simulink model "ofdmexample1"  (R2017a)
settings: Solver=FixedStepDiscrete  StartTime=0.0  StopTime=0.1  RelTol=1e-3
PostLoadFcn:
  | prm80216d.blkh = []; prm80216d.action = 'init';
  | commwman80216d_init(prm80216d.blkh, prm80216d.action);
  | if isempty(ans), clear ans; end
StartFcn:
  | if isempty(ans), clear ans; end
undefined symbols (not defined in the file): magnitude
libraries: commwman80216d_lib x25, dspsigops x8, commcnvcod2 x7, dspindex x4, commdigbbndpm3 x2, commblksprivate x1, commofdm x1, commsdrhw_v2 x1
Description:
  | IEEE 802.16-2004 WirelessMAN-OFDM PHY Downlink model
settings Model: FPTRunName=Active  ExtModeAutoUpdateStatusClock=off  Creator=The MathWorks, Inc.  LastModifiedBy=max
settings DataIOCC: LimitDataPoints=on  SaveFormat=Array
settings OptimizationCC: ExpressionDepthLimit=2147483647  InitFltsAndDblsToZero=on  EfficientMapNaN2IntZero=off  LifeSpan=inf
settings DebuggingCC: UnderspecifiedInitializationDetection=Classic  MergeDetectMultiDrivingBlocksExec=none  FcnCallInpInsideContextMsg=warning  AllowSymbolicDim=off  StateNameClashWarn=warning  SFUnexpectedBacktrackingDiag=warning  SFNoUnconditionalDefaultTransitionDiag=warning  SFExecutionAtInitializationDiag=none
settings HardwareCC: ProdBitPerPointer=32  ProdBitPerSizeT=32  ProdBitPerPtrDiffT=32  ProdLargestAtomicFloat=None  ProdIntDivRoundTo=Undefined  ProdEndianess=Unspecified  ProdWordSize=32  ProdHWDeviceType=32-bit Generic
settings ModelReferenceCC: PropagateSignalLabelsOutOfModel=off
settings RTWCC: RetainRTWFile=on
settings GRTTargetCC: TargetFcnLib=ansi_tfl_tmw_new.mat  TargetLangStandard=C89/C90 (ANSI)  GeneratePreprocessorConditionals=Disable all  CombineOutputUpdateFcns=off  GRTInterface=on
settings ConfigComp: CovMetricSettings=dw  CovHtmlReporting=on  CovSaveCumulativeToWorkspaceVar=on  CovSaveSingleToWorkspaceVar=on  CovExternalEMLEnable=off  CovSFcnEnable=off

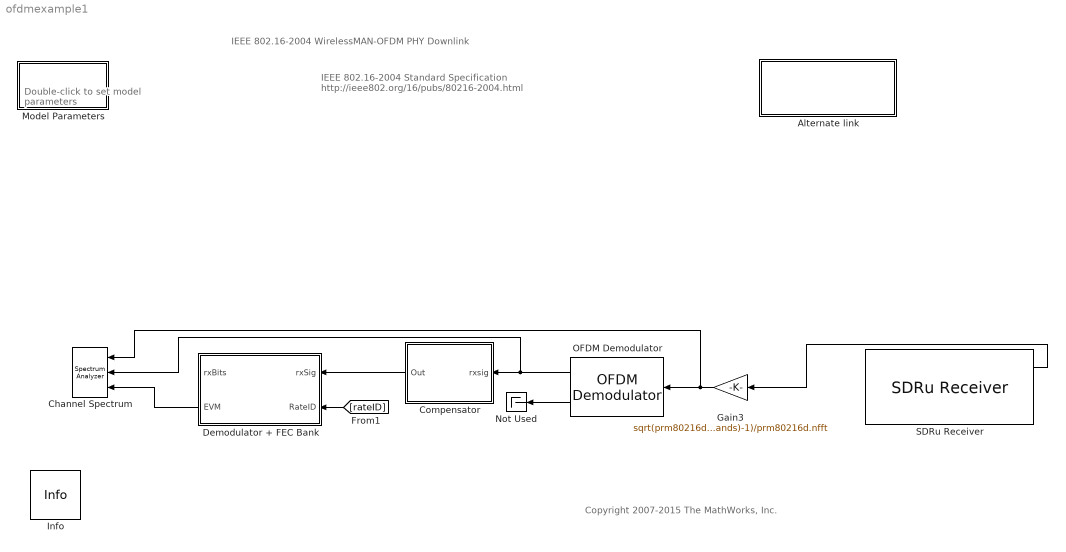
== system ofdmexample1 ==
  note: IEEE 802.16-2004 WirelessMAN-OFDM PHY Downlink
  note: Double-click to
      | set model parameters
  note: IEEE 802.16-2004 Standard Specification
      | http://ieee802.org/16/pubs/80216-2004.html
  note: Copyright 2007-2015 The MathWorks, Inc.
  Alternate link : Subsystem
      settings: OpenFcn=commwman80216dstbc;
      mask Display: disp('Double-click to open\n link model with\nSpace-Time Block Coding');
  Channel Spectrum : SpectrumAnalyzer  NumInputPorts=3
  Compensator : Subsystem
      mask Display: disp('Gain & Phase\nCompensator');
  Demodulator + FEC Bank : Subsystem
      mask Display: disp('Demodulator\n& FEC Bank');
  Gain3 : Gain  Gain=sqrt(prm80216d.nfft-sum(prm80216d.guardBands)-1)/prm80216d.nfft
  Info : commblksprivate/Info  SystemSampleTime=-1
      settings: SourceProductName=Communications System Toolbox  SourceProductBaseCode=CM
  Model Parameters : Subsystem  mask(Model Parameters){chanBW=3.5, numSym=1, g=1/8, nonlinCtrl=Disabled, dpdCtrl=Disabled, thresh=[4 10 12 19 22 28]}
      mask prompts: chanBW "Channel bandwidth (MHz):"; numSym "Number of OFDM symbols per burst:"; g "Cyclic prefix factor (G):"; nonlinCtrl "Amplifier nonlinearity:"; dpdCtrl "Digital pre-distortion:"; thresh "Low SNR thresholds for rate control (dB):"
      mask help: Specifies model parameters for a simulation run.
      mask init:
      | numPreSym = 1; % number of preamble OFDM symbols
      | 
      | % If the nonlinearity is turned off, then turn off the digital
      | % pre-distortion
      | if nonlinCtrl == 1  % disabled
      |     dpdCtrl = 1;
      | end
      | 
      | myException = commwman80216d_init(gcbh, 'init', chanBW, ...
      |     numSym, numPreSym, g, thresh);
      | 
      | if ~isempty(myException)
      |     errordlg(myException.msg);
      | end
      mask Help: helpview(commdhelp);
      mask TypeOptions g: 1/4 | 1/8 | 1/16 | 1/32
      mask TypeOptions nonlinCtrl: Disabled | Moderate (correctable by pre-distortion) | Severe (uncorrectable by pre-distortion)
      mask Callback nonlinCtrl: commwman80216d_init(gcbh, 'cbShowHidePreDistortion');
      mask TypeOptions dpdCtrl: Disabled | Enabled
      mask Display: disp('Model\nParameters');
  Not Used : Terminator
  OFDM Demodulator : commofdm/OFDM Demodulator  FFTLength=prm80216d.nfft  NumGuardBandCarriers=prm80216d.guardBands  RemoveDCCarrier=on  PilotOutputPort=on  PilotCarrierIndices=prm80216d.pilotIndices + prm80216d.nfft/2 + 1  CyclicPrefixLength=prm80216d.CPLen  NumSymbols=prm80216d.totOFDMSym  NumReceiveAntennas=1  SimulateUsing=Interpreted execution
      settings: SourceProductName=Communications System Toolbox  SourceProductBaseCode=CM
  SDRu Receiver : commsdrhw_v2/SDRu Receiver  SourceLibraryInfo="This block requires <a href=\"http://www.mathworks.com/hardware-support/usrp.html\">Communications System Toolbox Support Package for USRP Radio</a>"  rxtx=rx  platform=B210  USRP2_IP='192.168.10.2'  USRP_IP_X300='192.168.10.2'  USRP_IP_X310='192.168.10.2'  USRP_serialNumB200=''  USRP_serialNumB210='30D0D1D'  ChannelMapping=1  centerFrequency=2.484e9  centerFrequencySrc=Dialog  loOffset=0  loOffsetSrc=Dialog  PPSSource=Internal  clockSource=Internal  masterClkRateB200=32e6  masterClkRateB210=8e6  masterClkRateX300=200e6  masterClkRateX310=200e6  masterClkRateParam=8000000  gain=40  gainSrc=Dialog  decimInterpSrc=Dialog  decimInterp=512  TransportDataType=int16  USRP2_IP_NUM=[51 48 68 48 68 49 68]  frameLength=362  outputDatatype=Same as transport data type  overrunUnderrunPort=off  sampleTime=1/15625  HOST_DATA_PORT=0  HOST_CONTROL_PORT=0  USRP2_DATA_PORT=0  USRP2_CONTROL_PORT=0  bufferMode=Continuous streaming  EnableBurstMode=off  NumFramesInBurst=100  USRP_ID='30D0D1D'
      settings: SourceProductName=Communications System Toolbox Support Package for USRP(R) Radio  SourceProductBaseCode=USRP
  wires:
  [rateID] -> Demodulator + FEC Bank/2(RateID)
  Gain3/1 -> Channel Spectrum/1, OFDM Demodulator/1
  OFDM Demodulator/1 -> Channel Spectrum/2, Compensator/1(rxsig)
  OFDM Demodulator/2 -> Not Used/1
  Compensator/1(Out) -> Demodulator + FEC Bank/1(rxSig)
  Demodulator + FEC Bank/2(EVM) -> Channel Spectrum/3
  SDRu Receiver/1 -> Gain3/1

== system ofdmexample1/Alternate link ==

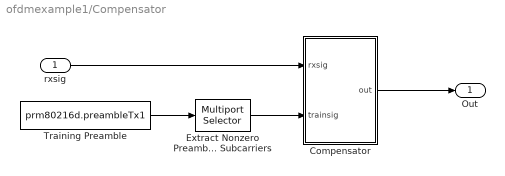
== system ofdmexample1/Compensator ==
  rxsig : Inport
  Compensator : Subsystem
      mask init:
      | a = [1:100; 1:100];
      mask Display: disp('Gain & Phase\nCompensator')
  Extract Nonzero Preamble Subcarriers : dspindex/Multiport Selector  rowsOrCols=Rows  idxCellArray=prm80216d.nonzeroPreambleIdxTx1  idxErrMode=Clip Index
  Training Preamble : Constant  Value=prm80216d.preambleTx1  VectorParams1D=off
  Out : Outport
  wires:
  Training Preamble/1 -> Extract Nonzero Preamble Subcarriers/1
  rxsig/1 -> Compensator/1(rxsig)
  Compensator/1(out) -> Out/1
  Extract Nonzero Preamble Subcarriers/1 -> Compensator/2(trainsig)

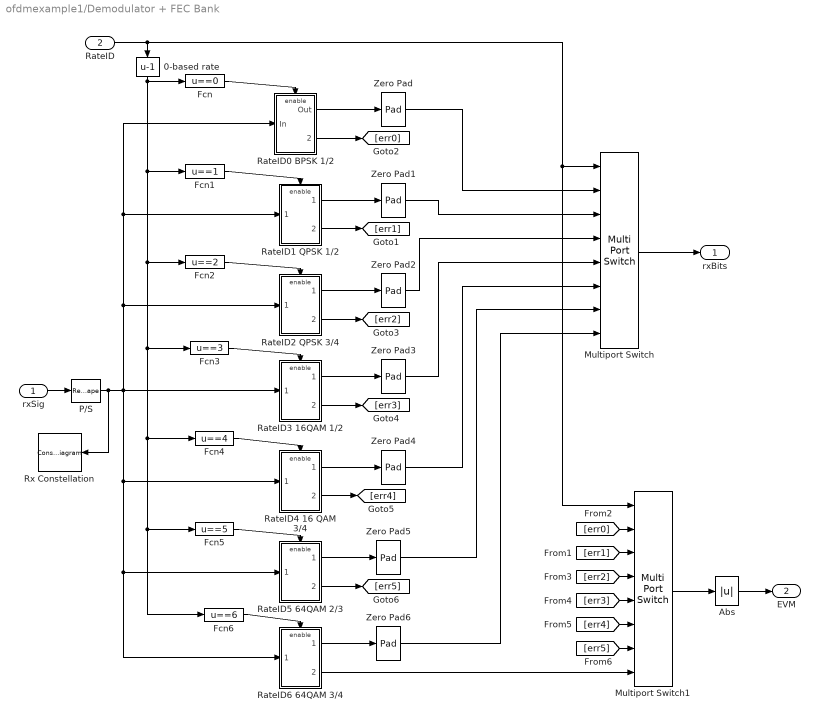
== system ofdmexample1/Demodulator + FEC Bank ==
  rxSig : Inport
  RateID : Inport  Port=2
  0-based rate : Bias  Bias=-1
  Abs : Abs  SaturateOnIntegerOverflow=on
  Fcn : Fcn  Expr=u==0
  Fcn1 : Fcn  Expr=u==1
  Fcn2 : Fcn  Expr=u==2
  Fcn3 : Fcn  Expr=u==3
  Fcn4 : Fcn  Expr=u==4
  Fcn5 : Fcn  Expr=u==5
  Fcn6 : Fcn  Expr=u==6
  Multiport Switch : MultiPortSwitch  Inputs=7  SaturateOnIntegerOverflow=on
  Multiport Switch1 : MultiPortSwitch  Inputs=7  SaturateOnIntegerOverflow=on
  P/S : Reshape  OutputDimensionality=Column vector (2-D)  OutputDimensions=[prm80216d.numDataSym, prm80216d.numOFDMSymbols]
  RateID0 BPSK 1/2 : Subsystem
  RateID1 QPSK 1/2 : Subsystem
  RateID2 QPSK 3/4 : Subsystem
  RateID3 16QAM 1/2 : Subsystem
  RateID4 16 QAM 3/4 : Subsystem
  RateID5 64QAM 2/3 : Subsystem
  RateID6 64QAM 3/4 : Subsystem
  Rx Constellation : ConstellationDiagram  Tag=ScatterPlot
  Zero Pad{,1..6} (7 alike) : dspsigops/Pad  padAlong=Columns  dimsToPad=1  valSrc=Specify via dialog  padVal=0  spec=Output size  padNumOutRowsSpecMethod=User-specified  numOutRows=prm80216d.maxUncBitsPerBlk*prm80216d.numOFDMSymbols  padNumOutColsSpecMethod=User-specified  numOutCols=1  isVarDimsMode=off  padBeginning=0  padEnd=0  outSizeMode=User-specified  outSize=1  padSigAt=End  trunc_flag=None  roundingMode=Floor  overflowMode=off  truncOrWrapMode=Truncate  wrap_flag=None
      settings: AttributesFormatString=\n  SourceProductName=DSP System Toolbox  SourceProductBaseCode=DS
  rxBits : Outport
  EVM : Outport  Port=2
  wires:
  RateID/1 -> Multiport Switch/1, Multiport Switch1/1, 0-based rate/1
  Multiport Switch/1 -> rxBits/1
  RateID0 BPSK 1/2/1(Out) -> Zero Pad/1
  RateID1 QPSK 1/2/1(Out1) -> Zero Pad1/1
  RateID2 QPSK 3/4/1(Out2) -> Zero Pad2/1
  RateID3 16QAM 1/2/1(Out3) -> Zero Pad3/1
  RateID4 16 QAM 3/4/1(Out4) -> Zero Pad4/1
  RateID5 64QAM 2/3/1(Out5) -> Zero Pad5/1
  RateID6 64QAM 3/4/1(Out6) -> Zero Pad6/1
  Fcn/1 -> RateID0 BPSK 1/2/Enable
  Fcn1/1 -> RateID1 QPSK 1/2/Enable
  Fcn2/1 -> RateID2 QPSK 3/4/Enable
  Fcn3/1 -> RateID3 16QAM 1/2/Enable
  Fcn4/1 -> RateID4 16 QAM 3/4/Enable
  Fcn5/1 -> RateID5 64QAM 2/3/Enable
  Fcn6/1 -> RateID6 64QAM 3/4/Enable
  Zero Pad/1 -> Multiport Switch/2
  Zero Pad2/1 -> Multiport Switch/4
  Zero Pad3/1 -> Multiport Switch/5
  Zero Pad4/1 -> Multiport Switch/6
  Zero Pad5/1 -> Multiport Switch/7
  Zero Pad6/1 -> Multiport Switch/8
  Multiport Switch1/1 -> Abs/1
  RateID6 64QAM 3/4/2(symerr) -> Multiport Switch1/8
  Abs/1 -> EVM/1
  0-based rate/1 -> Fcn/1, Fcn1/1, Fcn2/1, Fcn3/1, Fcn4/1, Fcn5/1, Fcn6/1
  RateID0 BPSK 1/2/2(symerr) -> [err0]
  RateID1 QPSK 1/2/2(symerr) -> [err1]
  RateID2 QPSK 3/4/2(symerr) -> [err2]
  RateID3 16QAM 1/2/2(symerr) -> [err3]
  RateID4 16 QAM 3/4/2(symerr) -> [err4]
  RateID5 64QAM 2/3/2(symerr) -> [err5]
  [err0] -> Multiport Switch1/2
  [err1] -> Multiport Switch1/3
  [err2] -> Multiport Switch1/4
  [err3] -> Multiport Switch1/5
  [err4] -> Multiport Switch1/6
  [err5] -> Multiport Switch1/7
  Zero Pad1/1 -> Multiport Switch/3
  rxSig/1 -> P/S/1
  P/S/1 -> Rx Constellation/1, RateID4 16 QAM 3/4/1(In4), RateID5 64QAM 2/3/1(In5), RateID6 64QAM 3/4/1(In6), RateID0 BPSK 1/2/1(In), RateID1 QPSK 1/2/1(In1), RateID2 QPSK 3/4/1(In2), RateID3 16QAM 1/2/1(In3)

== system ofdmexample1/Model Parameters ==
  note: This subsystem is empty.
      | It is used for setting parameter values (in the mask).

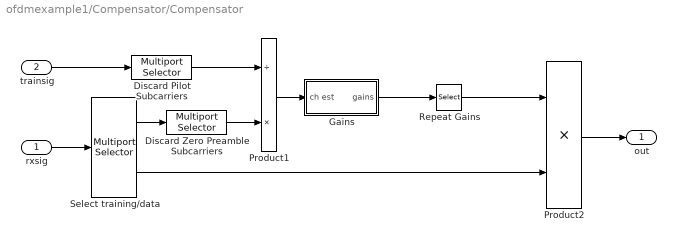
== system ofdmexample1/Compensator/Compensator ==
  rxsig : Inport
  trainsig : Inport  Port=2
  Discard Pilot Subcarriers : dspindex/Multiport Selector  rowsOrCols=Rows  idxCellArray=prm80216d.preambleEqIdxTx1  idxErrMode=Clip Index
  Discard Zero Preamble Subcarriers : dspindex/Multiport Selector  rowsOrCols=Rows  idxCellArray=prm80216d.dataEqIdxTx1  idxErrMode=Clip Index
  Gains : Subsystem
  Product1 : Product  Inputs=/*  SaturateOnIntegerOverflow=on  OutDataTypeStr=Inherit: Same as first input
  Product2 : Product  Inputs=**  SaturateOnIntegerOverflow=on  OutDataTypeStr=Inherit: Same as first input
  Repeat Gains : Selector  NumberOfDimensions=2  InputPortWidth=53  IndexOptions=Index vector (dialog),Select all  Indices=kron(1:prm80216d.numDataCarriers/2, [1 1]),-1  OutputSizes=1
  Select training/data : dspindex/Multiport Selector  rowsOrCols=Columns  idxCellArray={1:prm80216d.numPreamOFDMSymbols, prm80216d.numPreamOFDMSymbols+1:prm80216d.totOFDMSym}  idxErrMode=Clip Index
  out : Outport
  wires:
  Select training/data/1 -> Discard Zero Preamble Subcarriers/1
  Product2/1 -> out/1
  Product1/1 -> Gains/1(ch est)
  Gains/1(gains) -> Repeat Gains/1
  rxsig/1 -> Select training/data/1
  Repeat Gains/1 -> Product2/1
  Select training/data/2 -> Product2/2
  trainsig/1 -> Discard Pilot Subcarriers/1
  Discard Zero Preamble Subcarriers/1 -> Product1/2
  Discard Pilot Subcarriers/1 -> Product1/1

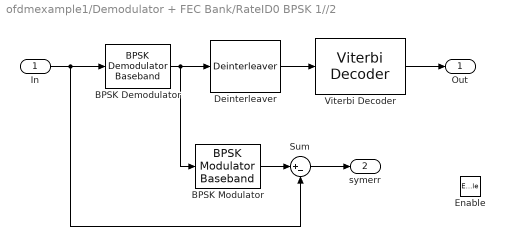
== system ofdmexample1/Demodulator + FEC Bank/RateID0 BPSK 1//2 ==
  In : Inport
  Enable : EnablePort  StatesWhenEnabling=reset  PropagateVarSize=During execution
  BPSK Demodulator : commdigbbndpm3/BPSK Demodulator Baseband  DecType=Hard decision  VarSource=Dialog  Variance=1  Ph=0  outDtype=boolean  derotateFactorWordLen=16  derotateFactorDataTypeStr=Inherit: Same word length as input  derotateFactorLastDataTypeStr=Inherit: Same word length as input
  BPSK Modulator : commdigbbndpm3/BPSK Modulator Baseband  Ph=0  outDtype=double  outWordLen=16  outUDDataType=sfix(16)  outFracLenMode=Best precision  outFracLen=15  outDataTypeStr=double  outLastDataTypeStr=double
  Deinterleaver : commwman80216d_lib/Deinterleaver  numSubCh=16  Ncbps1=192  Ncbps2=96  Ncbps3=48  Ncbps4=24  Ncbps5=12  Ncpc=1  numSym=prm80216d.numOFDMSymbols
      settings: SourceProductName=Communications System Toolbox  SourceProductBaseCode=CM
  Sum : Sum  Inputs=|+-  SaturateOnIntegerOverflow=on
  Viterbi Decoder : commcnvcod2/Viterbi Decoder  trellis=poly2trellis(7, [171 133])  isPunctured=off  punctureVector=reshape([1 0 1 0 1;1 1 0 1 0],10,1)  erasures=off  dectype=Hard decision  nsdecb=4  runSigValErrCheck=off  tbdepth=34  opmode=Truncated  reset=off  delayedResetAction=off  smWordLength=16  outDataType=boolean
      settings: SourceProductName=Communications System Toolbox  SourceProductBaseCode=CM
  Out : Outport
  symerr : Outport  Port=2  OutputWhenDisabled=reset  InitialOutput=0
  wires:
  Sum/1 -> symerr/1
  In/1 -> BPSK Demodulator/1, Sum/2
  BPSK Demodulator/1 -> Deinterleaver/1, BPSK Modulator/1
  Deinterleaver/1 -> Viterbi Decoder/1
  Viterbi Decoder/1 -> Out/1
  BPSK Modulator/1 -> Sum/1

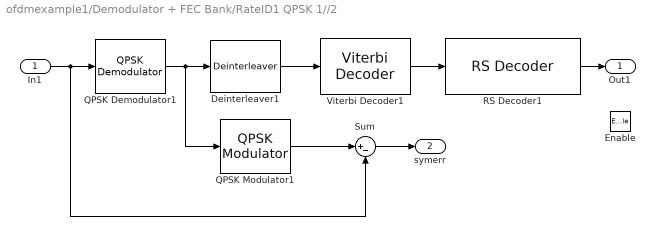
== system ofdmexample1/Demodulator + FEC Bank/RateID1 QPSK 1//2 ==
  In1 : Inport
  Enable : EnablePort  StatesWhenEnabling=reset  PropagateVarSize=During execution
  Deinterleaver1 : commwman80216d_lib/Deinterleaver  numSubCh=16  Ncbps1=384  Ncbps2=96  Ncbps3=48  Ncbps4=24  Ncbps5=12  Ncpc=2  numSym=prm80216d.numOFDMSymbols
      settings: SourceProductName=Communications System Toolbox  SourceProductBaseCode=CM
  QPSK Demodulator1 : commwman80216d_lib/QPSK Demodulator  SystemSampleTime=-1
      settings: SourceProductName=Communications System Toolbox  SourceProductBaseCode=CM
  QPSK Modulator1 : commwman80216d_lib/QPSK Modulator  SystemSampleTime=-1
      settings: SourceProductName=Communications System Toolbox  SourceProductBaseCode=CM
  RS Decoder1 : commwman80216d_lib/RS Decoder  N=32  K=24  numSym=prm80216d.numOFDMSymbols
      settings: SourceProductName=Communications System Toolbox  SourceProductBaseCode=CM
  Sum : Sum  Inputs=|+-  SaturateOnIntegerOverflow=on
  Viterbi Decoder1 : commcnvcod2/Viterbi Decoder  trellis=poly2trellis(7, [171 133])  isPunctured=on  punctureVector=reshape([1 0;1 1],4,1)  erasures=off  dectype=Hard decision  nsdecb=4  runSigValErrCheck=off  tbdepth=34  opmode=Truncated  reset=off  delayedResetAction=off  smWordLength=16  outDataType=boolean
      settings: SourceProductName=Communications System Toolbox  SourceProductBaseCode=CM
  Out1 : Outport
  symerr : Outport  Port=2  OutputWhenDisabled=reset  InitialOutput=0
  wires:
  In1/1 -> QPSK Demodulator1/1, Sum/2
  QPSK Demodulator1/1 -> Deinterleaver1/1, QPSK Modulator1/1
  Deinterleaver1/1 -> Viterbi Decoder1/1
  Viterbi Decoder1/1 -> RS Decoder1/1
  RS Decoder1/1 -> Out1/1
  Sum/1 -> symerr/1
  QPSK Modulator1/1 -> Sum/1

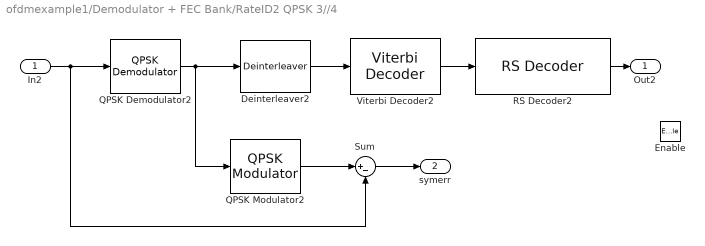
== system ofdmexample1/Demodulator + FEC Bank/RateID2 QPSK 3//4 ==
  In2 : Inport
  Enable : EnablePort  StatesWhenEnabling=reset  PropagateVarSize=During execution
  Deinterleaver2 : commwman80216d_lib/Deinterleaver  numSubCh=16  Ncbps1=384  Ncbps2=96  Ncbps3=48  Ncbps4=24  Ncbps5=12  Ncpc=2  numSym=prm80216d.numOFDMSymbols
      settings: SourceProductName=Communications System Toolbox  SourceProductBaseCode=CM
  QPSK Demodulator2 : commwman80216d_lib/QPSK Demodulator  SystemSampleTime=-1
      settings: SourceProductName=Communications System Toolbox  SourceProductBaseCode=CM
  QPSK Modulator2 : commwman80216d_lib/QPSK Modulator  SystemSampleTime=-1
      settings: SourceProductName=Communications System Toolbox  SourceProductBaseCode=CM
  RS Decoder2 : commwman80216d_lib/RS Decoder  N=40  K=36  numSym=prm80216d.numOFDMSymbols
      settings: SourceProductName=Communications System Toolbox  SourceProductBaseCode=CM
  Sum : Sum  Inputs=|+-  SaturateOnIntegerOverflow=on
  Viterbi Decoder2 : commcnvcod2/Viterbi Decoder  trellis=poly2trellis(7, [171 133])  isPunctured=on  punctureVector=reshape([1 0 1 0 1;1 1 0 1 0],10,1)  erasures=off  dectype=Hard decision  nsdecb=4  runSigValErrCheck=off  tbdepth=34  opmode=Truncated  reset=off  delayedResetAction=off  smWordLength=16  outDataType=boolean
      settings: SourceProductName=Communications System Toolbox  SourceProductBaseCode=CM
  Out2 : Outport
  symerr : Outport  Port=2  OutputWhenDisabled=reset  InitialOutput=0
  wires:
  In2/1 -> QPSK Demodulator2/1, Sum/2
  QPSK Demodulator2/1 -> Deinterleaver2/1, QPSK Modulator2/1
  Deinterleaver2/1 -> Viterbi Decoder2/1
  Viterbi Decoder2/1 -> RS Decoder2/1
  RS Decoder2/1 -> Out2/1
  QPSK Modulator2/1 -> Sum/1
  Sum/1 -> symerr/1

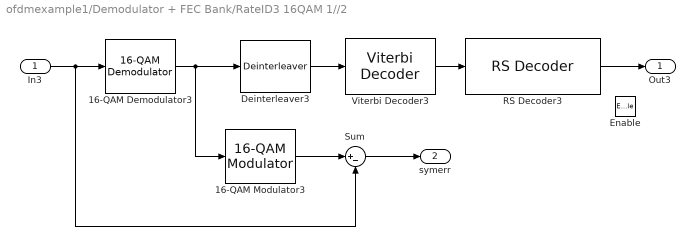
== system ofdmexample1/Demodulator + FEC Bank/RateID3 16QAM 1//2 ==
  In3 : Inport
  Enable : EnablePort  StatesWhenEnabling=reset  PropagateVarSize=During execution
  16-QAM Demodulator3 : commwman80216d_lib/16-QAM Demodulator  SystemSampleTime=-1
      settings: SourceProductName=Communications System Toolbox  SourceProductBaseCode=CM
  16-QAM Modulator3 : commwman80216d_lib/16-QAM Modulator  SystemSampleTime=-1
      settings: SourceProductName=Communications System Toolbox  SourceProductBaseCode=CM
  Deinterleaver3 : commwman80216d_lib/Deinterleaver  numSubCh=16  Ncbps1=768  Ncbps2=96  Ncbps3=48  Ncbps4=24  Ncbps5=12  Ncpc=4  numSym=prm80216d.numOFDMSymbols
      settings: SourceProductName=Communications System Toolbox  SourceProductBaseCode=CM
  RS Decoder3 : commwman80216d_lib/RS Decoder  N=64  K=48  numSym=prm80216d.numOFDMSymbols
      settings: SourceProductName=Communications System Toolbox  SourceProductBaseCode=CM
  Sum : Sum  Inputs=|+-  SaturateOnIntegerOverflow=on
  Viterbi Decoder3 : commcnvcod2/Viterbi Decoder  trellis=poly2trellis(7, [171 133])  isPunctured=on  punctureVector=reshape([1 0;1 1],4,1)  erasures=off  dectype=Hard decision  nsdecb=4  runSigValErrCheck=off  tbdepth=34  opmode=Truncated  reset=off  delayedResetAction=off  smWordLength=16  outDataType=boolean
      settings: SourceProductName=Communications System Toolbox  SourceProductBaseCode=CM
  Out3 : Outport
  symerr : Outport  Port=2  OutputWhenDisabled=reset  InitialOutput=0
  wires:
  In3/1 -> 16-QAM Demodulator3/1, Sum/2
  16-QAM Demodulator3/1 -> Deinterleaver3/1, 16-QAM Modulator3/1
  Deinterleaver3/1 -> Viterbi Decoder3/1
  Viterbi Decoder3/1 -> RS Decoder3/1
  RS Decoder3/1 -> Out3/1
  16-QAM Modulator3/1 -> Sum/1
  Sum/1 -> symerr/1

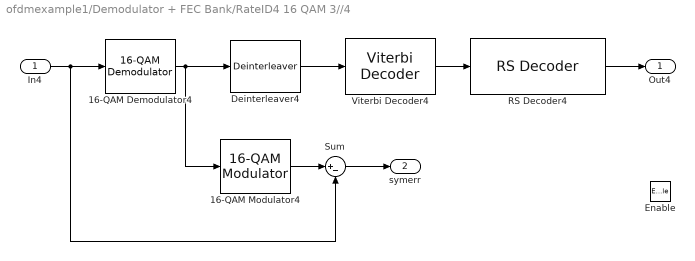
== system ofdmexample1/Demodulator + FEC Bank/RateID4 16 QAM 3//4 ==
  In4 : Inport
  Enable : EnablePort  StatesWhenEnabling=reset  PropagateVarSize=During execution
  16-QAM Demodulator4 : commwman80216d_lib/16-QAM Demodulator  SystemSampleTime=-1
      settings: SourceProductName=Communications System Toolbox  SourceProductBaseCode=CM
  16-QAM Modulator4 : commwman80216d_lib/16-QAM Modulator  SystemSampleTime=-1
      settings: SourceProductName=Communications System Toolbox  SourceProductBaseCode=CM
  Deinterleaver4 : commwman80216d_lib/Deinterleaver  numSubCh=16  Ncbps1=768  Ncbps2=96  Ncbps3=48  Ncbps4=24  Ncbps5=12  Ncpc=4  numSym=prm80216d.numOFDMSymbols
      settings: SourceProductName=Communications System Toolbox  SourceProductBaseCode=CM
  RS Decoder4 : commwman80216d_lib/RS Decoder  N=80  K=72  numSym=prm80216d.numOFDMSymbols
      settings: SourceProductName=Communications System Toolbox  SourceProductBaseCode=CM
  Sum : Sum  Inputs=|+-  SaturateOnIntegerOverflow=on
  Viterbi Decoder4 : commcnvcod2/Viterbi Decoder  trellis=poly2trellis(7, [171 133])  isPunctured=on  punctureVector=reshape([1 0 1 0 1;1 1 0 1 0],10,1)  erasures=off  dectype=Hard decision  nsdecb=4  runSigValErrCheck=off  tbdepth=34  opmode=Truncated  reset=off  delayedResetAction=off  smWordLength=16  outDataType=boolean
      settings: SourceProductName=Communications System Toolbox  SourceProductBaseCode=CM
  Out4 : Outport
  symerr : Outport  Port=2  OutputWhenDisabled=reset  InitialOutput=0
  wires:
  In4/1 -> 16-QAM Demodulator4/1, Sum/2
  16-QAM Demodulator4/1 -> Deinterleaver4/1, 16-QAM Modulator4/1
  Deinterleaver4/1 -> Viterbi Decoder4/1
  Viterbi Decoder4/1 -> RS Decoder4/1
  RS Decoder4/1 -> Out4/1
  Sum/1 -> symerr/1
  16-QAM Modulator4/1 -> Sum/1

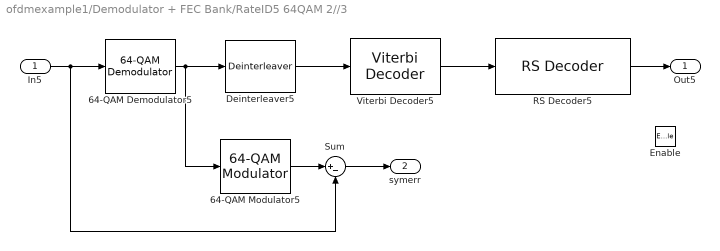
== system ofdmexample1/Demodulator + FEC Bank/RateID5 64QAM 2//3 ==
  In5 : Inport
  Enable : EnablePort  StatesWhenEnabling=reset  PropagateVarSize=During execution
  64-QAM Demodulator5 : commwman80216d_lib/64-QAM Demodulator  SystemSampleTime=-1
      settings: SourceProductName=Communications System Toolbox  SourceProductBaseCode=CM
  64-QAM Modulator5 : commwman80216d_lib/64-QAM Modulator  SystemSampleTime=-1
      settings: SourceProductName=Communications System Toolbox  SourceProductBaseCode=CM
  Deinterleaver5 : commwman80216d_lib/Deinterleaver  numSubCh=16  Ncbps1=1152  Ncbps2=96  Ncbps3=48  Ncbps4=24  Ncbps5=12  Ncpc=6  numSym=prm80216d.numOFDMSymbols
      settings: SourceProductName=Communications System Toolbox  SourceProductBaseCode=CM
  RS Decoder5 : commwman80216d_lib/RS Decoder  N=108  K=96  numSym=prm80216d.numOFDMSymbols
      settings: SourceProductName=Communications System Toolbox  SourceProductBaseCode=CM
  Sum : Sum  Inputs=|+-  SaturateOnIntegerOverflow=on
  Viterbi Decoder5 : commcnvcod2/Viterbi Decoder  trellis=poly2trellis(7, [171 133])  isPunctured=on  punctureVector=reshape([1 0 1;1 1 0 ],6,1)  erasures=off  dectype=Hard decision  nsdecb=4  runSigValErrCheck=off  tbdepth=34  opmode=Truncated  reset=off  delayedResetAction=off  smWordLength=16  outDataType=boolean
      settings: SourceProductName=Communications System Toolbox  SourceProductBaseCode=CM
  Out5 : Outport
  symerr : Outport  Port=2  OutputWhenDisabled=reset  InitialOutput=0
  wires:
  In5/1 -> 64-QAM Demodulator5/1, Sum/2
  64-QAM Demodulator5/1 -> Deinterleaver5/1, 64-QAM Modulator5/1
  Deinterleaver5/1 -> Viterbi Decoder5/1
  Viterbi Decoder5/1 -> RS Decoder5/1
  RS Decoder5/1 -> Out5/1
  Sum/1 -> symerr/1
  64-QAM Modulator5/1 -> Sum/1

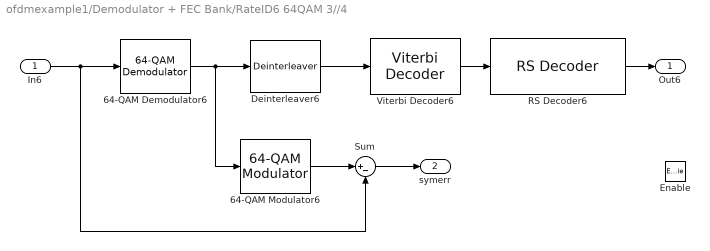
== system ofdmexample1/Demodulator + FEC Bank/RateID6 64QAM 3//4 ==
  In6 : Inport
  Enable : EnablePort  StatesWhenEnabling=reset  PropagateVarSize=During execution
  64-QAM Demodulator6 : commwman80216d_lib/64-QAM Demodulator  SystemSampleTime=-1
      settings: SourceProductName=Communications System Toolbox  SourceProductBaseCode=CM
  64-QAM Modulator6 : commwman80216d_lib/64-QAM Modulator  SystemSampleTime=-1
      settings: SourceProductName=Communications System Toolbox  SourceProductBaseCode=CM
  Deinterleaver6 : commwman80216d_lib/Deinterleaver  numSubCh=16  Ncbps1=1152  Ncbps2=96  Ncbps3=48  Ncbps4=24  Ncbps5=12  Ncpc=6  numSym=prm80216d.numOFDMSymbols
      settings: SourceProductName=Communications System Toolbox  SourceProductBaseCode=CM
  RS Decoder6 : commwman80216d_lib/RS Decoder  N=120  K=108  numSym=prm80216d.numOFDMSymbols
      settings: SourceProductName=Communications System Toolbox  SourceProductBaseCode=CM
  Sum : Sum  Inputs=|+-  SaturateOnIntegerOverflow=on
  Viterbi Decoder6 : commcnvcod2/Viterbi Decoder  trellis=poly2trellis(7, [171 133])  isPunctured=on  punctureVector=reshape([1 0 1 0 1;1 1 0 1 0], 10, 1)  erasures=off  dectype=Hard decision  nsdecb=4  runSigValErrCheck=off  tbdepth=34  opmode=Truncated  reset=off  delayedResetAction=off  smWordLength=16  outDataType=boolean
      settings: SourceProductName=Communications System Toolbox  SourceProductBaseCode=CM
  Out6 : Outport
  symerr : Outport  Port=2  OutputWhenDisabled=reset  InitialOutput=0
  wires:
  In6/1 -> 64-QAM Demodulator6/1, Sum/2
  64-QAM Demodulator6/1 -> Deinterleaver6/1, 64-QAM Modulator6/1
  Deinterleaver6/1 -> Viterbi Decoder6/1
  Viterbi Decoder6/1 -> RS Decoder6/1
  RS Decoder6/1 -> Out6/1
  Sum/1 -> symerr/1
  64-QAM Modulator6/1 -> Sum/1

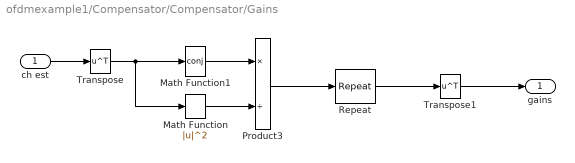
== system ofdmexample1/Compensator/Compensator/Gains ==
  ch est : Inport
  Math Function : Math  Operator=magnitude^2  SaturateOnIntegerOverflow=on
  Math Function1 : Math  Operator=conj  SaturateOnIntegerOverflow=on
  Product3 : Product  Inputs=*/  SaturateOnIntegerOverflow=on  OutDataTypeStr=Inherit: Same as first input
  Repeat : dspsigops/Repeat  N=prm80216d.numOFDMSymbols  InputProcessing=Columns as channels (frame based)  RateOptions=Enforce single-rate processing  ic=0  mode=Unused parameter value
      settings: SourceProductName=DSP System Toolbox
  Transpose : Math  Operator=transpose  SaturateOnIntegerOverflow=on
  Transpose1 : Math  Operator=transpose  SaturateOnIntegerOverflow=on
  gains : Outport
  wires:
  Product3/1 -> Repeat/1
  Transpose1/1 -> gains/1
  Repeat/1 -> Transpose1/1
  Transpose/1 -> Math Function/1, Math Function1/1
  Math Function1/1 -> Product3/1
  Math Function/1 -> Product3/2
  ch est/1 -> Transpose/1
